simulink model "ex1_pid_simulink"  (R2023b)
settings: Solver=FixedStepAuto  StartTime=0.0  StopTime=10  FixedStep=Ts  RelTol=1e-3
InitFcn:
  | params
values from neighbouring files (symbols this model uses):
  J = 0.02    [motor_ex.m]    (also in params.m)
  Kb = 0.1    [motor_ex.m]    (also in params.m)
  KD = 0.5    [ex1_pid.m]    (also in params.m)
  Kf = 0.2    [motor_ex.m]    (also in params.m = 0.01)
  KI = 0.1    [ex1_pid.m]    (also in params.m)
  Km = 0.1    [motor_ex.m]    (also in params.m = 1)
  KP = 0.7    [ex1_pid.m]    (also in params.m)
  L = 0.5    [motor_ex.m]    (also in params.m)
  R = 2.0    (= 2)    [motor_ex.m]    (also in params.m)
settings Model: Creator=SJ  LastModifiedBy=SJ

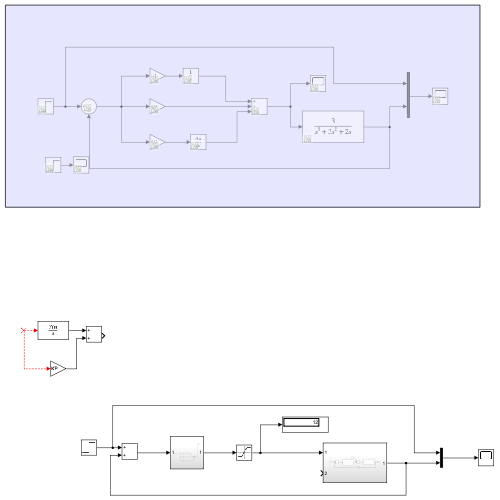
[thumbnail: Simulink's stored preview of the top-level diagram]
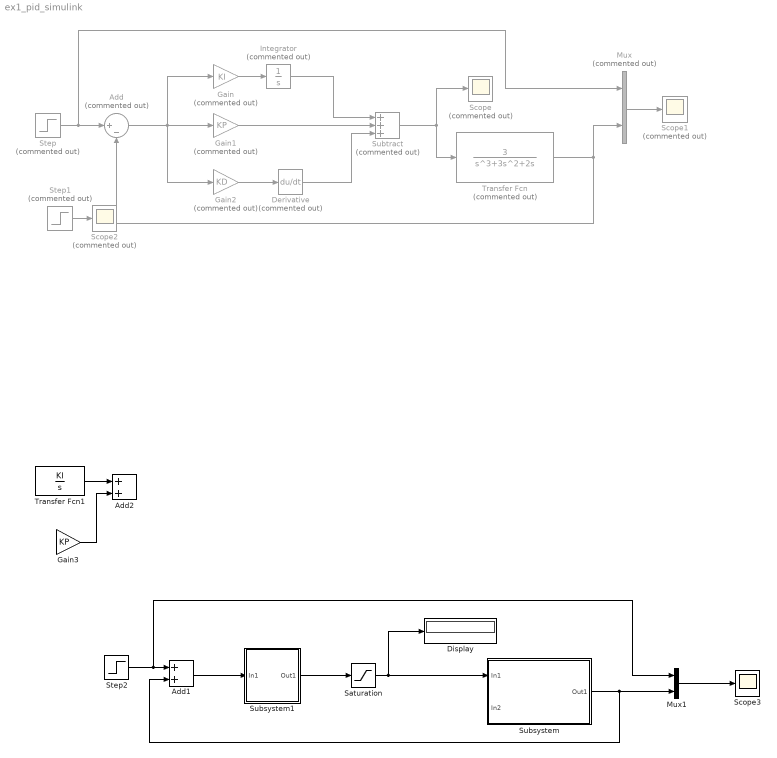
== system ex1_pid_simulink ==
  Add : Sum  Commented=on  Inputs=|+-
  Add1 : Sum
  Add2 : Sum
  Derivative : Derivative  Commented=on
  Display : Display
  Gain : Gain  Commented=on  Gain=KI
  Gain1 : Gain  Commented=on  Gain=KP
  Gain2 : Gain  Commented=on  Gain=KD
  Gain3 : Gain  Gain=KP
  Integrator : Integrator  Commented=on
  Mux : Mux  Commented=on  Inputs=2
  Mux1 : Mux  Inputs=2
  Saturation : Saturate  UpperLimit=12  LowerLimit=0
  Scope : Scope  Commented=on
  Scope1 : Scope  Commented=on
  Scope2 : Scope  Commented=on
  Scope3 : Scope
  Step : Step  Commented=on  SampleTime=0
  Step1 : Step  Commented=on  SampleTime=0
  Step2 : Step  After=100  SampleTime=0
  Subsystem : Subsystem
  Subsystem1 : Subsystem
  Subtract : Sum  Commented=on  Inputs=+++
  Transfer Fcn : TransferFcn  Commented=on  Numerator=3  Denominator=[1 3 2 0]
  Transfer Fcn1 : TransferFcn  Numerator=KI  Denominator=[1 0]
  wires:
  Mux/1 -> Scope1/1
  Transfer Fcn/1 -> Mux/2, Add/2
  Gain/1 -> Integrator/1
  Integrator/1 -> Subtract/1
  Derivative/1 -> Subtract/3
  Gain1/1 -> Subtract/2
  Gain2/1 -> Derivative/1
  Add/1 -> Gain/1, Gain2/1, Gain1/1
  Subtract/1 -> Scope/1, Transfer Fcn/1
  Step/1 -> Mux/1, Add/1
  Step1/1 -> Scope2/1
  Step2/1 -> Mux1/1, Add1/1
  Saturation/1 -> Display/1, Subsystem/1(In1)
  Subsystem/1(Out1) -> Add1/2, Mux1/2
  Mux1/1 -> Scope3/1
  ? -> Gain3/1
  ? -> Transfer Fcn1/1
  Transfer Fcn1/1 -> Add2/1
  Gain3/1 -> Add2/2
  Subsystem1/1(Out1) -> Saturation/1
  Add1/1 -> Subsystem1/1(In1)

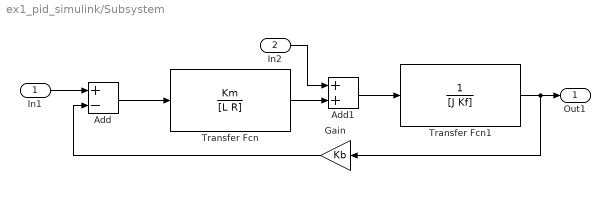
== system ex1_pid_simulink/Subsystem ==
  In1 : Inport
  In2 : Inport  Port=2
  Add : Sum  Inputs=+-
  Add1 : Sum
  Gain : Gain  Gain=Kb
  Transfer Fcn : TransferFcn  Numerator=Km  Denominator=[L R]
  Transfer Fcn1 : TransferFcn  Numerator=1  Denominator=[J Kf]
  Out1 : Outport
  wires:
  In1/1 -> Add/1
  In2/1 -> Add1/1
  Add/1 -> Transfer Fcn/1
  Add1/1 -> Transfer Fcn1/1
  Transfer Fcn/1 -> Add1/2
  Gain/1 -> Add/2
  Transfer Fcn1/1 -> Gain/1, Out1/1

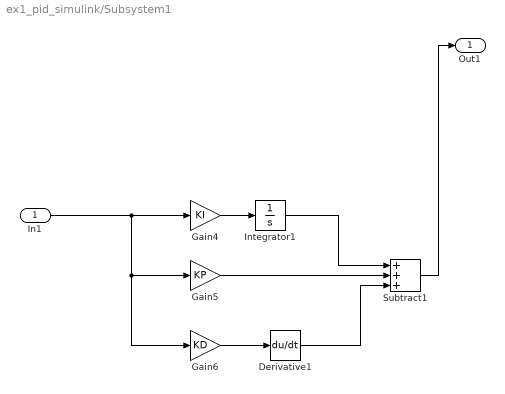
== system ex1_pid_simulink/Subsystem1 ==
  In1 : Inport
  Derivative1 : Derivative
  Gain4 : Gain  Gain=KI
  Gain5 : Gain  Gain=KP
  Gain6 : Gain  Gain=KD
  Integrator1 : Integrator
  Subtract1 : Sum  Inputs=+++
  Out1 : Outport
  wires:
  Subtract1/1 -> Out1/1
  In1/1 -> Gain5/1, Gain6/1, Gain4/1
  Integrator1/1 -> Subtract1/1
  Derivative1/1 -> Subtract1/3
  Gain6/1 -> Derivative1/1
  Gain5/1 -> Subtract1/2
  Gain4/1 -> Integrator1/1
